simulink model "Events3Out"  (Simulink 5.0)
settings: Solver=ode45  StartTime=0.0  StopTime=10.0  RelTol=1e-3
settings Model: Creator=scaife  LastModifiedBy=scaife  ExtModeAutoUpdateStatusClock=off

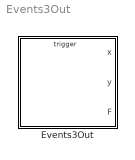
== system Events3Out ==
  Events3Out : Stateflow chart

== stateflow chart Events3Out ==
  state TOP1 [parallel]
    state A/
      en: x+=10;
    state B/
      en:x+=1000;
    (default) -> A : {x++;}
    A -> B : G{x+=100;}/E;
    B -> A : G{x+=100;}/E;
  state TOP2 [parallel]
    state C/
      en: y+=10;
    state D/
      en: y+=1000;
    (default) -> C : {y++;}
    C -> D : E{y+=100;}/F;
    D -> C : E{y+=100;}/F;
  data: x output int32; y output int32
  events: E local EITHER_EDGE_EVENT; F output FUNCTION_CALL_EVENT; G input RISING_EDGE_EVENT
